simulink model "Prac6_Simu_AHM"  (R2025b)
settings: Solver=VariableStepAuto  StartTime=0.0  StopTime=0.01  MaxStep=0.00001  RelTol=1e-3
InitFcn:
  | L = 2e-3;
  | C = 10e-6;
  | R = 10;
  | Uin = 32;

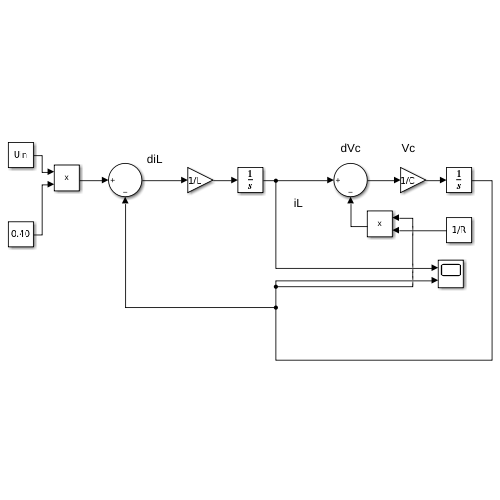
[thumbnail: Simulink's stored preview of the top-level diagram]
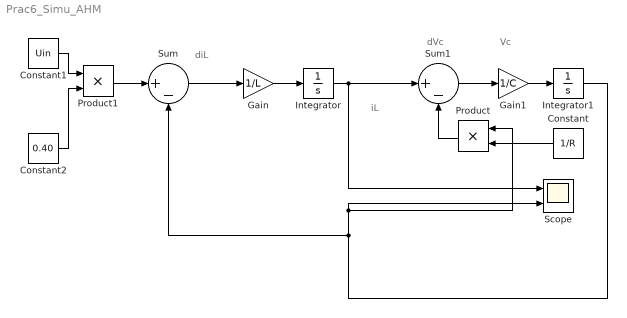
== system Prac6_Simu_AHM ==
  note: Vc
  note: dVc
  note: iL
  note: diL
  Constant : Constant  Value=1/R
  Constant1 : Constant  Value=Uin
  Constant2 : Constant  Value=0.40
  Gain : Gain  Gain=1/L
  Gain1 : Gain  Gain=1/C
  Integrator : Integrator
  Integrator1 : Integrator
  Product : Product
  Product1 : Product
  Scope : Scope  NumInputPorts=2
      settings: ActiveDisplayYMinimum=-1.6691218158068881  ActiveDisplayYMaximum=15.022096342261998
  Sum : Sum  Inputs=|+-
  Sum1 : Sum  Inputs=|+-
  wires:
  Integrator/1 -> Scope/1, Sum1/1
  Integrator1/1 -> Product/1, Scope/2, Sum/2
  Sum/1 -> Gain/1
  Gain/1 -> Integrator/1
  Gain1/1 -> Integrator1/1
  Sum1/1 -> Gain1/1
  Constant/1 -> Product/2
  Product/1 -> Sum1/2
  Product1/1 -> Sum/1
  Constant1/1 -> Product1/1
  Constant2/1 -> Product1/2
